simulink model "controller"  (R2016b)
settings: Solver=FixedStepDiscrete  StartTime=0.0  StopTime=10.0  FixedStep=0.1  RelTol=1e-3
undefined symbols (not defined in the file): BaseDrag, FireRocketHeight, GravityConstant, Mass, OpenChuteHeight
settings Model: Creator=csax  LastModifiedBy=csax
settings OptimizationCC: DefaultParameterBehavior=Inlined
settings DebuggingCC: ParameterTunabilityLossMsg=error
settings HardwareCC: ProdBitPerPointer=32  ProdBitPerSizeT=32  ProdBitPerPtrDiffT=32  ProdLargestAtomicFloat=None  ProdWordSize=32  ProdHWDeviceType=Custom Processor->Custom
settings RTWCC: SystemTargetFile=trace32_target_ert.tlc  MakeCommand=trace32_target_make  TemplateMakefile=trace32_arm_tmf.tmf  Description=TRACE32 Target  GenerateReport=on  IncludeHyperlinkInReport=on  LaunchReport=on  GenerateTraceInfo=on  GenerateTraceReport=on  GenerateTraceReportSl=on  GenerateTraceReportSf=on  GenerateTraceReportEml=on
settings CodeAppCC: ForceParamTrailComments=on  IgnoreCustomStorageClasses=off  OperatorAnnotations=on  SimulinkDataObjDesc=on  SFDataObjDesc=on  MATLABFcnDesc=on  InsertBlockDesc=on  MATLABSourceComments=on
settings STFCustomTargetCC: TargetLangStandard=C99 (ISO)  CombineOutputUpdateFcns=on  ERTCustomFileBanners=on  SupportContinuousTime=off  SupportNonInlinedSFcns=off  RemoveResetFunc=on  MATLABClassNameForMDSCustomization=Simulink.SoftwareTarget.ERTCustomization  GRTInterface=off  SystemTargetFile=trace32_target_ert.tlc
settings ERTTargetCC: TargetLangStandard=C99 (ISO)  ParMdlRefBuildCompliant=off  CompOptLevelCompliant=off  ConcurrentExecutionCompliant=off  ERTFirstTimeCompliant=off  ModelStepFunctionPrototypeControlCompliant=off  CPPClassGenCompliant=off  UseToolchainInfoCompliant=off  InlinedParameterPlacement=NonHierarchical  ERTCustomFileTemplate=example_file_process.tlc

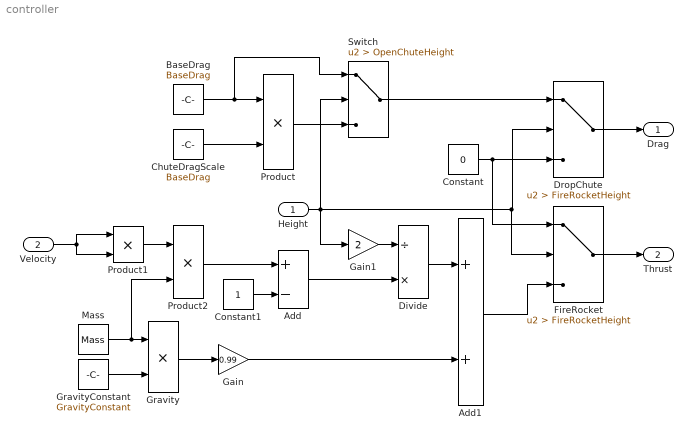
== system controller ==
  Height : Inport
  Velocity : Inport  Port=2
  Add : Sum  Inputs=+-
  Add1 : Sum
  BaseDrag : Constant  Value=BaseDrag
  ChuteDragScale : Constant  Value=BaseDrag
  Constant : Constant  Value=0
  Constant1 : Constant
  Divide : Product  Inputs=/*
  DropChute : Switch  Criteria=u2 > Threshold  Threshold=FireRocketHeight
  FireRocket : Switch  Criteria=u2 > Threshold  Threshold=FireRocketHeight
  Gain : Gain  Gain=0.99
  Gain1 : Gain  Gain=2
  Gravity : Product
  GravityConstant : Constant  Value=GravityConstant
  Mass : Constant  Value=Mass
  Product : Product
  Product1 : Product
  Product2 : Product
  Switch : Switch  Criteria=u2 > Threshold  Threshold=OpenChuteHeight
  Drag : Outport
  Thrust : Outport  Port=2
  wires:
  Switch/1 -> DropChute/1
  DropChute/1 -> Drag/1
  Constant/1 -> FireRocket/1, DropChute/3
  FireRocket/1 -> Thrust/1
  GravityConstant/1 -> Gravity/2
  Mass/1 -> Product2/2, Gravity/1
  Gravity/1 -> Gain/1
  Product1/1 -> Product2/1
  Product2/1 -> Add/1
  Constant1/1 -> Add/2
  Add/1 -> Divide/2
  Gain1/1 -> Divide/1
  Divide/1 -> Add1/1
  Gain/1 -> Add1/2
  BaseDrag/1 -> Product/1, Switch/1
  Product/1 -> Switch/3
  ChuteDragScale/1 -> Product/2
  Add1/1 -> FireRocket/3
  Velocity/1 -> Product1/2, Product1/1
  Height/1 -> Gain1/1, FireRocket/2, DropChute/2, Switch/2
